simulink model "qam_model"  (R2013a)
settings: Solver=ode45  StartTime=0.0  StopTime=4e5*Tclk  RelTol=1e-3
PreLoadFcn:
  | crec_init;
StopFcn:
  | %offset = 70000;
  | % figure; u=sd(offset:end,:);plot(u(:,1)+j*u(:,2), '.');
values from neighbouring files (symbols this model uses):
  Fadc = 50    [qam_init.m]
  qam_mode = 2    [qam_init.m]
  Tclk = 1/Fclk    (= 0.01)    [qam_init.m]
undefined symbols (not defined in the file or in its folder): A, get, N
libraries: xbsIndex_r4 x29, commsink2 x7, dspsigops x3, dspsrcs4 x2, PPEthernetRuntimeCosim_r4 x1
settings Model: Creator=alexp  LastModifiedBy=diego
settings DataIOCC: MaxDataPoints=10000  SignalLoggingSaveFormat=ModelDataLogs
settings OptimizationCC: BooleanDataType=off  ExpressionDepthLimit=2147483647
settings DebuggingCC: SaveWithParameterizedLinksMsg=none  SignalResolutionControl=TryResolveAllWithWarning  SolverPrmCheckMsg=none  MultiTaskDSMMsg=warning  MultiTaskCondExecSysMsg=none  FcnCallInpInsideContextMsg=UseLocalSettings  StrictBusMsg=None
settings HardwareCC: TargetUnknown=on
settings RTWCC: IncludeERTFirstTime=on
settings GRTTargetCC: CombineOutputUpdateFcns=off  GRTInterface=on

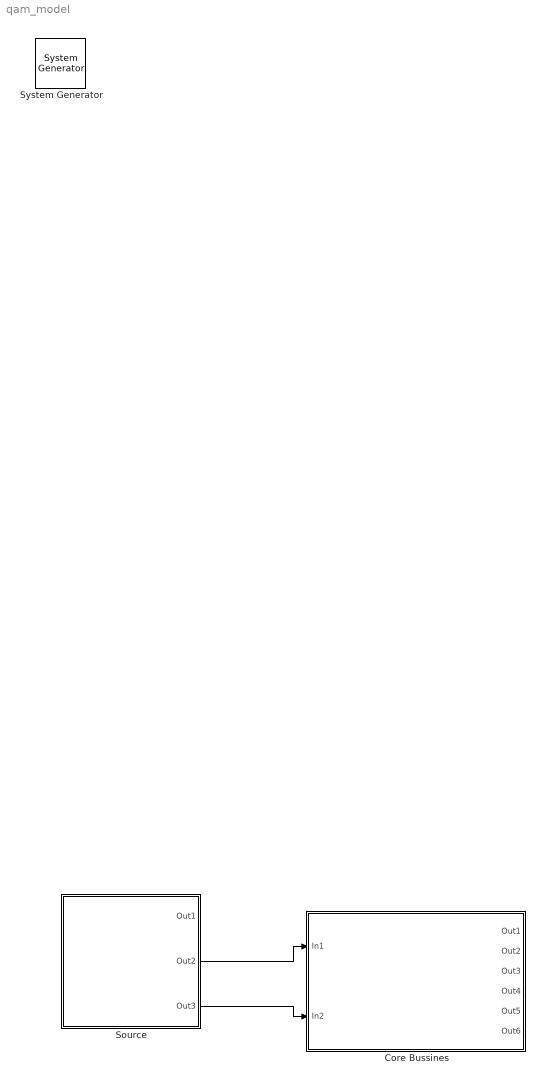
== system qam_model ==
  " System Generator" : xbsIndex_r4/ System Generator  Tag=genX  xilinxfamily=spartan6  part=xc6slx45t  speed=-3  package=fgg484  synthesis_tool=XST  clock_wrapper=Clock Enables  directory=./netlist  proj_type=Project Navigator  Synth_file=XST Defaults  Impl_file=ISE Defaults  testbench=off  simulink_period=Tclk  sysclk_period=20  dcm_input_clock_period=10  incr_netlist=off  trim_vbits=Everywhere in SubSystem  dbl_ovrd=According to Block Masks  core_generation=According to Block Masks  run_coregen=off  deprecated_control=off  eval_field=0  block_type=sysgen
  Core Bussines : Subsystem
  Source : Subsystem
  wires:
  Source/2(Out2) -> Core Bussines/1(In1)
  Source/3(Out3) -> Core Bussines/2(In2)

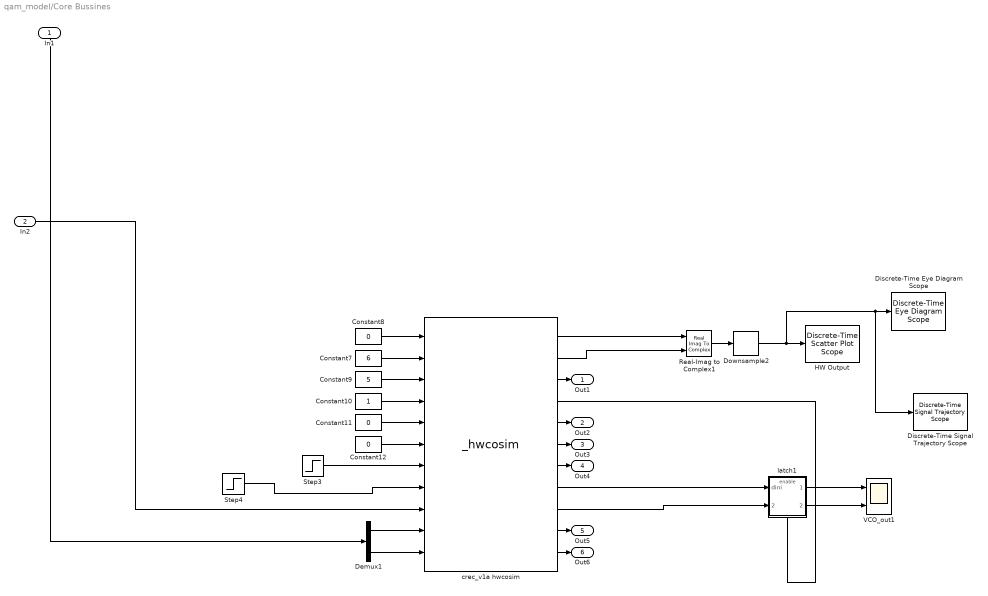
== system qam_model/Core Bussines ==
  In1 : Inport
  In2 : Inport  Port=2
  Constant10 : Constant
  Constant11 : Constant  Value=0
  Constant12 : Constant  Value=0
  Constant7 : Constant  Value=6
  Constant8 : Constant  Value=0
  Constant9 : Constant  Value=5
  Demux1 : Demux  Outputs=2
  Discrete-Time Eye Diagram Scope : commsink2/Discrete-Time Eye Diagram Scope  Tag=EyeDiagram  sampPerSymb=8  offsetEye=0  symbPerTrace=1  numTraces=800  numNewFrames=800  LineStyles=-  LineColors=[1 0 1]  dupPoints=on  fading=on  render=on  AxisGrid=on  yMin=-0.368939208984375  yMax=0.366009521484375  inphaseLabel=In-phase Amplitude  quadratureLabel=Quadrature Amplitude  openScopeAtSimStart=on  dispDiagram=In-phase and Quadrature  FrameNumber=off  FigPos=get(0,'defaultfigureposition');  figTitle=Eye Diagram  block_type_=eye  numLinesMax=8
  Discrete-Time Signal Trajectory Scope : commsink2/Discrete-Time Signal Trajectory Scope  Tag=SignalTrajectory  sampPerSymb=8  offsetEye=0  numTraces=800  numNewFrames=800  LineStyles=-  LineColors=b  fading=on  render=on  AxisGrid=on  xMin=-0.367013549804688  xMax=0.366525268554688  yMin=-0.368905639648438  yMax=0.364633178710938  inphaseLabel=In-phase Amplitude  quadratureLabel=Quadrature Amplitude  openScopeAtSimStart=on  FrameNumber=off  FigPos=get(0,'defaultfigureposition');  figTitle=Signal Trajectory  numLinesMax=8  block_type_=xy
  Downsample2 : dspsigops/Downsample  N=4  phase=0  InputProcessing=Columns as channels (frame based)  RateOptions=Allow multirate processing  smode=Allow multirate  fmode=Maintain input frame size  ic=0
  HW Output : commsink2/Discrete-Time Scatter Plot Scope  Tag=ScatterPlot  sampPerSymb=1  offsetEye=0  numTraces=2^qam_mode*1000  numNewFrames=2^qam_mode*200  LineMarkers=.  LineColors=[1 0 0]  fading=on  render=on  AxisGrid=on  xMin=-0.361343383789062  xMax=0.357070922851562  yMin=-0.360366821289062  yMax=0.358047485351562  inphaseLabel=In-phase Amplitude  quadratureLabel=Quadrature Amplitude  openScopeAtSimStart=on  FrameNumber=off  FigPos=get(0,'defaultfigureposition');  figTitle=Scatter Plot  numLinesMax=8  block_type_=scatter
  Real-Imag to Complex1 : RealImagToComplex
  Step3 : Step  Time=20*Tclk  Before=1  After=0  SampleTime=Tclk
  Step4 : Step  Time=100*Tclk  Before=1  After=0  SampleTime=Tclk
  VCO_out1 : Scope  NumInputPorts=2
      settings: YMin=-1~-1  YMax=1~1  SaveName=aa
  crec_v1a hwcosim : PPEthernetRuntimeCosim_r4/_hwcosim  clkSrc=Single Stepped  hasCombinationalPath=on  bitfileName=/home/diego/qam_demudulator/mirror/xapp1173/netlist/crec_v1a_cw.bit  ethernetInterface=Please select an Ethernet interface  fpgaEthernetAddr=00:0a:35:11:22:33  cable=Auto Detect  speed=N/A  cablePort=N/A  configTimeout=3000  configProfile=Default settings  enable_codebug=on  design_xtable=|  cosim_xtable=|  ethernetInterfaceID=eth0  timeout=3000  useWaitBox=1  prgClkFreq=10  bscanPos=1  Scheme=Cosim  hasProc=0  skipConfig=0  block_type=ppethernet_cosim
      design_xtable=|
      | {
      |   'clkWrapper' => 'crec_v1a_cw',
      |   'clocksGcd' => 1,
      |   'device' => 'xc6slx45t-3fgg484',
      |   'ports' => {
      |     'cnotrol' => {
      |       'bd_port_index' => 0,
      |       'direction' => 'in',
      |       'icon_text' => 'cnotrol',
      |       'period' => 1,
      |       'sim_pause_trigger' => false,
      |       'type' => 'UFix_2_0',
      |       'width' => 2,
      |     },
      |     'cnotrol1' => {
      |       'bd_port_index' => 1,
      |       'direction' => 'in',
      |       'icon_text' => 'cnotrol1',
      |       'period' => 1,
      |       'sim_pause_trigger' => false,
      |       'type' => 'Fix_8_0',
      |       'width' => 8,
      |     },
      |     'cnotrol2' => {
      |       'bd_port_index' => 2,
      |       'direction' => 'in',
      |       'icon_text' => 'cnotrol2',
      |       'period' => 1,
      |       'sim_pause_trigger' => false,
      |       'type' => 'Fix_8_0',
      |       'width' => 8,
      |     },
      |     'cnotrol3' => {
      |       'bd_port_index' => 3,
      |       'direction' => 'in',
      |       'icon_text' => 'cnotrol3',
      |       'period' => 1,
      |       'sim_pause_trigger' => false,
      |       'type' => 'Fix_8_0',
      |       'width' => 8,
      |     },
      |     'cnotrol4' => {
      |       'bd_port_index' => 4,
      |       'direction' => 'in',
      |       'icon_text' => 'cnotrol4',
      |       'period' => 1,
      |       'sim_pause_trigger' => false,
      |       'type' => 'UFix_1_0',
      |       'width' => 1,
      |     },
      |     'cnotrol5' => {
      |       'bd_port_index' => 5,
      |       'direction' => 'in',
      |       'icon_text' => 'cnotrol5',
      |       'period' => 1,
      |       'sim_pause_trigger' => false,
      |       'type' => 'Fix_28_26',
      |       'width' => 28,
      |     },
      |     'cnotrol6' => {
      |       'bd_port_index' => 6,
      |       'direction' => 'in',
      |       'icon_text' => 'cnotrol6',
      |       'period' => 1,
      |       'sim_pause_trigger' => false,
      |       'type' => 'Bool',
      |       'width' => 1,
      |     },
      |     'cnotrol7' => {
      |       'bd_port_index' => 7,
      |       'direction' => 'in',
      |       'icon_text' => 'cnotrol7',
      |       'period' => 1,
      |       'sim_pause_trigger' => false,
      |       'type' => 'Bool',
      |       'width' => 1,
      |     },
      |     'cnotrol8' => {
      |       'bd_port_index' => 8,
      |       'direction' => 'in',
      |       'icon_text' => 'cnotrol8',
      |       'period' => 1,
      |       'sim_pause_trigger' => false,
      |       'type' => 'Bool',
      |       'width' => 1,
      |     },
      |     'din_i' => {
      |       'bd_port_index' => 9,
      |       'direction' => 'in',
      |       'icon_text' => 'din_i',
      |       'period' => 1,
      |       'sim_pause_trigger' => false,
      |       'type' => 'Fix_16_13',
      |       'width' => 16,
      |     },
      |     'din_q' => {
      |       'bd_port_index' => 10,
      |       'direction' => 'in',
      |       'icon_text' => 'din_q',
      |       'period' => 1,
      |       'sim_pause_trigger' => false,
      |       'type' => 'Fix_16_13',
      |       'width' => 16,
      |     },
      |     'gateway_out' => {
      |       'bd_port_index' => 0,
      |       'direction' => 'out',
      |       'icon_text' => 'Gateway Out',
      |       'period' => 1,
      |       'sim_pause_trigger' => false,
      |       'type' => 'Fix_16_13',
      |       'width' => 16,
      |     },
      |     'gateway_out1' => {
      |       'bd_port_index' => 1,
      |       'direction' => 'out',
      |       'icon_text' => 'Gateway Out1',
      |       'period' => 1,
      |       'sim_pause_trigger' => false,
      |       'type' => 'Fix_16_13',
      |       'width' => 16,
      |     },
      |     'gateway_out10' => {
      |       'bd_port_index' => 2,
      |       'direction' => 'out',
      |       'icon_text' => 'Gateway Out10',
      |       'period' => 1,
      |       'sim_pause_trigger' => false,
      |       'type' => 'Fix_12_11',
      |       'width' => 12,
      |     },
      |     'gateway_out2' => {
      |       'bd_port_index' => 3,
      |       'direction' => 'out',
      |       'icon_text' => 'Gateway Out2',
      |       'period' => 1,
      |       'sim_pause_trigger' => false,
      |       'type' => 'Bool',
      |       'width' => 1,
      |     },
      |     'gateway_out3' => {
      |       'bd_port_index' => 4,
      |       'direction' => 'out',
      |       'icon_text' => 'Gateway Out3',
      |       'period' => 1,
      |       'sim_pause_trigger' => false,
      |       'type' => 'Fix_28_26',
      |       'width' => 28,
      |     },
      |     'gateway_out4' => {
      |       'bd_port_index' => 5,
      |       'direction' => 'out',
      |       'icon_text' => 'Gateway Out4',
      |       'period' => 1,
      |       'sim_pause_trigger' => false,
      |       'type' => 'Bool',
      |       'width' => 1,
      |     },
      |     'gateway_out5' => {
      |       'bd_port_index' => 6,
      |       'direction' => 'out',
      |       'icon_text' => 'Gateway Out5',
      |       'period' => 1,
      |       'sim_pause_trigger' => false,
      |       'type' => 'Bool',
      |       'width' => 1,
      |     },
      |     'gateway_out6' => {
      |       'bd_port_index' => 7,
      |       'direction' => 'out',
      |       'icon_text' => 'Gateway Out6',
      |       'period' => 1,
      |       'sim_pause_trigger' => false,
      |       'type' => 'Fix_12_11',
      |       'width' => 12,
      |     },
      |     'gateway_out7' => {
      |       'bd_port_index' => 8,
      |       'direction' => 'out',
      |       'icon_text' => 'Gateway Out7',
      |       'period' => 1,
      |       'sim_pause_trigger' => false,
      |       'type' => 'Fix_12_11',
      |       'width' => 12,
      |     },
      |     'gateway_out8' => {
      |       'bd_port_index' => 9,
      |       'direction' => 'out',
      |       'icon_text' => 'Gateway Out8',
      |       'period' => 1,
      |       'sim_pause_trigger' => false,
      |       'type' => 'Bool',
      |       'width' => 1,
      |     },
      |     'gateway_out9' => {
      |       'bd_port_index' => 10,
      |       'direction' => 'out',
      |       'icon_text' => 'Gateway Out9',
      |       'period' => 1,
      |       'sim_pause_trigger' => false,
      |       'type' => 'Fix_12_11',
      |       'width' => 12,
      |     },
      |   },
      |   'shared_memories' => {},
      | }
      cosim_xtable=|
      | {
      |   'ethernetCosim' => {
      |     'blockRAMSize' => 2048,
      |     'bscanPos' => 2,
      |     'maxFrameSize' => 8184,
      |     'target' => 'sp605',
      |     'type' => 'ppethernet',
      |   },
      | }
  latch1 : Subsystem  TreatAsAtomicUnit=on
  Out1 : Outport
  Out2 : Outport  Port=2
  Out3 : Outport  Port=3
  Out4 : Outport  Port=4
  Out5 : Outport  Port=5
  Out6 : Outport  Port=6
  wires:
  Step3/1 -> crec_v1a hwcosim/7
  Step4/1 -> crec_v1a hwcosim/8
  Demux1/2 -> crec_v1a hwcosim/11
  Demux1/1 -> crec_v1a hwcosim/10
  Downsample2/1 -> Discrete-Time Signal Trajectory Scope/1, Discrete-Time Eye Diagram Scope/1, HW Output/1
  Real-Imag to Complex1/1 -> Downsample2/1
  crec_v1a hwcosim/8 -> latch1/1(dini)
  crec_v1a hwcosim/2 -> Real-Imag to Complex1/2
  crec_v1a hwcosim/1 -> Real-Imag to Complex1/1
  crec_v1a hwcosim/10 -> Out5/1
  crec_v1a hwcosim/7 -> Out4/1
  crec_v1a hwcosim/5 -> Out2/1
  In1/1 -> Demux1/1
  Constant11/1 -> crec_v1a hwcosim/5
  In2/1 -> crec_v1a hwcosim/9
  Constant8/1 -> crec_v1a hwcosim/1
  Constant9/1 -> crec_v1a hwcosim/3
  Constant10/1 -> crec_v1a hwcosim/4
  crec_v1a hwcosim/6 -> Out3/1
  crec_v1a hwcosim/11 -> Out6/1
  crec_v1a hwcosim/3 -> Out1/1
  crec_v1a hwcosim/4 -> latch1/Enable
  latch1/2(doutq) -> VCO_out1/2
  crec_v1a hwcosim/9 -> latch1/2(dinq)
  latch1/1(douti) -> VCO_out1/1
  Constant12/1 -> crec_v1a hwcosim/6
  Constant7/1 -> crec_v1a hwcosim/2

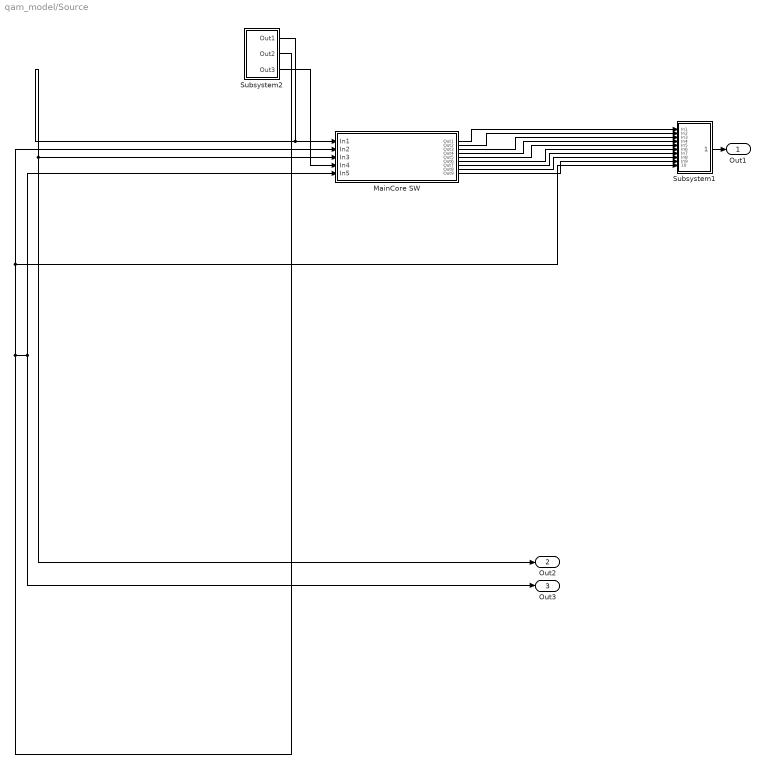
== system qam_model/Source ==
  MainCore SW : Subsystem
  Subsystem1 : Subsystem
  Subsystem2 : Subsystem
  Out1 : Outport
  Out2 : Outport  Port=2
  Out3 : Outport  Port=3
  wires:
  Subsystem2/3(Out3) -> MainCore SW/4(In4)
  Subsystem1/1(Out1) -> Out1/1
  MainCore SW/5(Out5) -> Subsystem1/5(In5)
  MainCore SW/3(Out3) -> Subsystem1/3(In3)
  Subsystem2/2(Out2) -> MainCore SW/2(In2), Subsystem1/10(In10), Out3/1, MainCore SW/5(In5)
  MainCore SW/8(Out8) -> Subsystem1/8(In8)
  MainCore SW/2(Out2) -> Subsystem1/2(In2)
  MainCore SW/4(Out4) -> Subsystem1/4(In4)
  Subsystem2/1(Out1) -> Out2/1, MainCore SW/3(In3), MainCore SW/1(In1)
  MainCore SW/9(Out9) -> Subsystem1/9(In9)
  MainCore SW/6(Out6) -> Subsystem1/6(In6)
  MainCore SW/7(Out7) -> Subsystem1/7(In7)
  MainCore SW/1(Out1) -> Subsystem1/1(In1)

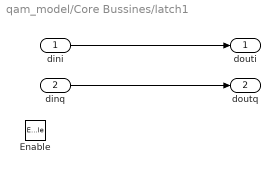
== system qam_model/Core Bussines/latch1 ==
  dini : Inport
  dinq : Inport  Port=2
  Enable : EnablePort
  douti : Outport
  doutq : Outport  Port=2
  wires:
  dini/1 -> douti/1
  dinq/1 -> doutq/1

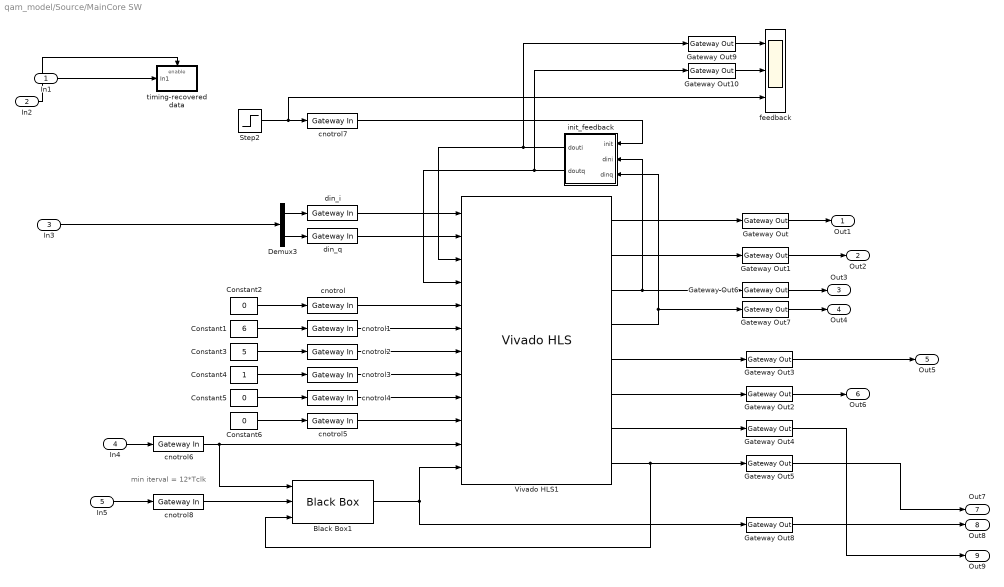
== system qam_model/Source/MainCore SW ==
  note: min iterval = 12*Tclk
  In1 : Inport
  In2 : Inport  Port=2
  In3 : Inport  Port=3
  In4 : Inport  Port=4
  In5 : Inport  Port=5
  Black Box1 : xbsIndex_r4/Black Box  init_code=start_config  sim_method=ISE Simulator  verbose=off  block_type=blackbox2
  Constant1 : Constant  Value=6
  Constant2 : Constant  Value=0
  Constant3 : Constant  Value=5
  Constant4 : Constant
  Constant5 : Constant  Value=0
  Constant6 : Constant  Value=0
  Demux3 : Demux  Outputs=2
  Gateway Out{,1..10} (11 alike) : xbsIndex_r4/Gateway Out  inherit_from_input=off  hdl_port=on  timing_constraint=None  locs_specified=off  LOCs={}  UseAsDAC=off  DACChannel='1'  block_type=gatewayout
  Step2 : Step  Time=100*Tclk  Before=1  After=0  SampleTime=Tclk
  Vivado HLS1 : xbsIndex_r4/Vivado HLS  anytable='/home/diego/qam_demudulator/mirror/xapp1173/VHLS_proj/sol3_dataflow_io/'  display_datatype=off  rate_propagation_method=Simulink system period  model_file_path=''  latency=1  block_type=hls
      settings: infoedit=This block allows including C,C++ and SystemC source files in System Generator for DSP designs.
  cnotrol : xbsIndex_r4/Gateway In  gui_display_data_type=Fixed-point  arith_type=Unsigned  n_bits=2  bin_pt=0  preci_type=Single  exp_width=8  frac_width=24  quantization=Truncate  overflow=Wrap  period=Tclk  dbl_ovrd=off  timing_constraint=None  locs_specified=off  LOCs={}  UseAsADC=off  ADCChannel='1'  inherit_from_input=off  hdl_port=on  block_type=gatewayin
  cnotrol1 : xbsIndex_r4/Gateway In  gui_display_data_type=Fixed-point  arith_type="Signed  (2's comp)"  n_bits=8  bin_pt=0  preci_type=Single  exp_width=8  frac_width=24  quantization=Truncate  overflow=Wrap  period=Tclk  dbl_ovrd=off  timing_constraint=None  locs_specified=off  LOCs={}  UseAsADC=off  ADCChannel='1'  inherit_from_input=off  hdl_port=on  block_type=gatewayin
  cnotrol2 : xbsIndex_r4/Gateway In  gui_display_data_type=Fixed-point  arith_type="Signed  (2's comp)"  n_bits=8  bin_pt=0  preci_type=Single  exp_width=8  frac_width=24  quantization=Truncate  overflow=Wrap  period=Tclk  dbl_ovrd=off  timing_constraint=None  locs_specified=off  LOCs={}  UseAsADC=off  ADCChannel='1'  inherit_from_input=off  hdl_port=on  block_type=gatewayin
  cnotrol3 : xbsIndex_r4/Gateway In  gui_display_data_type=Fixed-point  arith_type="Signed  (2's comp)"  n_bits=8  bin_pt=0  preci_type=Single  exp_width=8  frac_width=24  quantization=Truncate  overflow=Wrap  period=Tclk  dbl_ovrd=off  timing_constraint=None  locs_specified=off  LOCs={}  UseAsADC=off  ADCChannel='1'  inherit_from_input=off  hdl_port=on  block_type=gatewayin
  cnotrol4 : xbsIndex_r4/Gateway In  gui_display_data_type=Fixed-point  arith_type=Unsigned  n_bits=1  bin_pt=0  preci_type=Single  exp_width=8  frac_width=24  quantization=Truncate  overflow=Wrap  period=Tclk  dbl_ovrd=off  timing_constraint=None  locs_specified=off  LOCs={}  UseAsADC=off  ADCChannel='1'  inherit_from_input=off  hdl_port=on  block_type=gatewayin
  cnotrol5 : xbsIndex_r4/Gateway In  gui_display_data_type=Fixed-point  arith_type="Signed  (2's comp)"  n_bits=28  bin_pt=26  preci_type=Single  exp_width=8  frac_width=24  quantization=Truncate  overflow=Wrap  period=Tclk  dbl_ovrd=off  timing_constraint=None  locs_specified=off  LOCs={}  UseAsADC=off  ADCChannel='1'  inherit_from_input=off  hdl_port=on  block_type=gatewayin
  cnotrol6 : xbsIndex_r4/Gateway In  gui_display_data_type=Boolean  arith_type=Boolean  n_bits=2  bin_pt=0  preci_type=Single  exp_width=8  frac_width=24  quantization=Truncate  overflow=Wrap  period=Tclk  dbl_ovrd=off  timing_constraint=None  locs_specified=off  LOCs={}  UseAsADC=off  ADCChannel='1'  inherit_from_input=off  hdl_port=on  block_type=gatewayin
  cnotrol7 : xbsIndex_r4/Gateway In  gui_display_data_type=Boolean  arith_type=Boolean  n_bits=2  bin_pt=0  preci_type=Single  exp_width=8  frac_width=24  quantization=Truncate  overflow=Wrap  period=Tclk  dbl_ovrd=off  timing_constraint=None  locs_specified=off  LOCs={}  UseAsADC=off  ADCChannel='1'  inherit_from_input=off  hdl_port=on  block_type=gatewayin
  cnotrol8 : xbsIndex_r4/Gateway In  gui_display_data_type=Boolean  arith_type=Boolean  n_bits=2  bin_pt=0  preci_type=Single  exp_width=8  frac_width=24  quantization=Truncate  overflow=Wrap  period=Tclk  dbl_ovrd=off  timing_constraint=None  locs_specified=off  LOCs={}  UseAsADC=off  ADCChannel='1'  inherit_from_input=off  hdl_port=on  block_type=gatewayin
  din_i : xbsIndex_r4/Gateway In  gui_display_data_type=Fixed-point  arith_type="Signed  (2's comp)"  n_bits=16  bin_pt=13  preci_type=Single  exp_width=8  frac_width=24  quantization=Truncate  overflow=Wrap  period=Tclk  dbl_ovrd=off  timing_constraint=None  locs_specified=off  LOCs={}  UseAsADC=off  ADCChannel='1'  inherit_from_input=off  hdl_port=on  block_type=gatewayin
  din_q : xbsIndex_r4/Gateway In  gui_display_data_type=Fixed-point  arith_type="Signed  (2's comp)"  n_bits=16  bin_pt=13  preci_type=Single  exp_width=8  frac_width=24  quantization=Truncate  overflow=Wrap  period=Tclk  dbl_ovrd=off  timing_constraint=None  locs_specified=off  LOCs={}  UseAsADC=off  ADCChannel='1'  inherit_from_input=off  hdl_port=on  block_type=gatewayin
  feedback : Scope  NumInputPorts=3
      settings: YMin=-1~-1~-5  YMax=1~1~5  SaveName=aa1
  init_feedback : Subsystem
  timing-recovered data : Subsystem  TreatAsAtomicUnit=on
  Out1 : Outport
  Out2 : Outport  Port=2
  Out3 : Outport  Port=3
  Out4 : Outport  Port=4
  Out5 : Outport  Port=5
  Out6 : Outport  Port=6
  Out7 : Outport  Port=7
  Out8 : Outport  Port=8
  Out9 : Outport  Port=9
  wires:
  In5/1 -> cnotrol8/1
  In2/1 -> timing-recovered data/Enable
  In1/1 -> timing-recovered data/1(In1)
  Constant3/1 -> cnotrol2/1
  Constant2/1 -> cnotrol/1
  Constant1/1 -> cnotrol1/1
  Constant4/1 -> cnotrol3/1
  Constant5/1 -> cnotrol4/1
  Constant6/1 -> cnotrol5/1
  In4/1 -> cnotrol6/1
  Demux3/2 -> din_q/1
  Demux3/1 -> din_i/1
  Gateway Out3/1 -> Out5/1
  cnotrol/1 -> Vivado HLS1/5
  cnotrol1/1 -> Vivado HLS1/6
  cnotrol2/1 -> Vivado HLS1/7
  cnotrol3/1 -> Vivado HLS1/8
  cnotrol4/1 -> Vivado HLS1/9
  cnotrol5/1 -> Vivado HLS1/10
  cnotrol6/1 -> Vivado HLS1/11, Black Box1/1
  din_i/1 -> Vivado HLS1/1
  din_q/1 -> Vivado HLS1/2
  Vivado HLS1/1 -> Gateway Out/1
  Vivado HLS1/2 -> Gateway Out1/1
  Vivado HLS1/5 -> Gateway Out3/1
  Vivado HLS1/6 -> Gateway Out2/1
  Vivado HLS1/7 -> Gateway Out4/1
  Vivado HLS1/8 -> Gateway Out5/1, Black Box1/3
  Gateway Out4/1 -> Out9/1
  cnotrol8/1 -> Black Box1/2
  Black Box1/1 -> Vivado HLS1/12, Gateway Out8/1
  Gateway Out2/1 -> Out6/1
  Gateway Out/1 -> Out1/1
  Gateway Out1/1 -> Out2/1
  Gateway Out5/1 -> Out7/1
  init_feedback/1(douti) -> Gateway Out9/1, Vivado HLS1/3
  init_feedback/2(doutq) -> Gateway Out10/1, Vivado HLS1/4
  Vivado HLS1/4 -> init_feedback/3(dinq), Gateway Out7/1
  Vivado HLS1/3 -> init_feedback/2(dini), Gateway Out6/1
  Step2/1 -> cnotrol7/1, feedback/3
  cnotrol7/1 -> init_feedback/1(init)
  Gateway Out6/1 -> Out3/1
  Gateway Out7/1 -> Out4/1
  Gateway Out8/1 -> Out8/1
  Gateway Out9/1 -> feedback/1
  Gateway Out10/1 -> feedback/2
  In3/1 -> Demux3/1

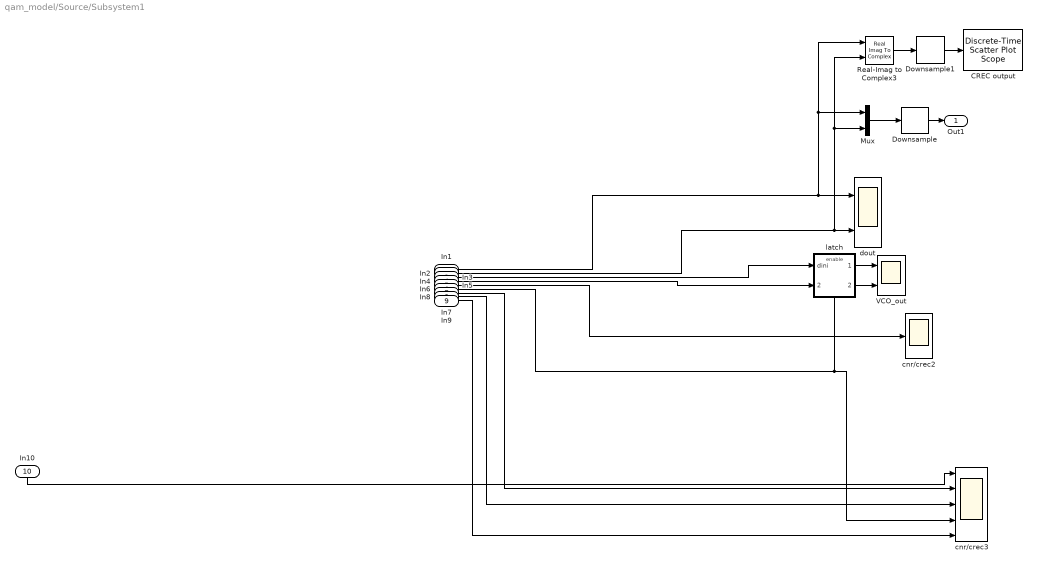
== system qam_model/Source/Subsystem1 ==
  In1 : Inport
  In2 : Inport  Port=2
  In3 : Inport  Port=3
  In4 : Inport  Port=4
  In5 : Inport  Port=5
  In6 : Inport  Port=6
  In7 : Inport  Port=7
  In8 : Inport  Port=8
  In9 : Inport  Port=9
  In10 : Inport  Port=10
  CREC output : commsink2/Discrete-Time Scatter Plot Scope  Tag=ScatterPlot  sampPerSymb=1  offsetEye=0  numTraces=2^qam_mode*1000  numNewFrames=2^qam_mode*200  LineMarkers=.  LineColors=b  fading=on  render=on  AxisGrid=on  xMin=-1.2  xMax=1.2  yMin=-1.2  yMax=1.2  inphaseLabel=In-phase Amplitude  quadratureLabel=Quadrature Amplitude  openScopeAtSimStart=on  FrameNumber=off  FigPos=get(0,'defaultfigureposition');  figTitle=Scatter Plot  numLinesMax=8  block_type_=scatter
  Downsample : dspsigops/Downsample  N=4  phase=0  InputProcessing=Columns as channels (frame based)  RateOptions=Allow multirate processing  smode=Allow multirate  fmode=Maintain input frame size  ic=0
  Downsample1 : dspsigops/Downsample  N=4  phase=0  InputProcessing=Columns as channels (frame based)  RateOptions=Allow multirate processing  smode=Allow multirate  fmode=Maintain input frame size  ic=0
  Mux : Mux  Inputs=2
  Real-Imag to Complex3 : RealImagToComplex
  VCO_out : Scope  NumInputPorts=2
      settings: YMin=-1~-1  YMax=1~1  SaveName=aa9
  cnr/crec2 : Scope
      settings: TimeRange=4000  YMin=-0.0012  YMax=0.0004  SaveName=aa6  Decimation=32
  cnr/crec3 : Scope  NumInputPorts=5
      settings: YMin=0~0~0~0~0  YMax=1.2~1.1~1.2~1.2~1.2  SaveName=aa7
  dout : Scope  NumInputPorts=2
      settings: YMin=-0.4~-0.4  YMax=0.4~0.4  SaveName=aa8
  latch : Subsystem  TreatAsAtomicUnit=on
  Out1 : Outport
  wires:
  In2/1 -> dout/2, Mux/2, Real-Imag to Complex3/2
  In1/1 -> Mux/1, Real-Imag to Complex3/1, dout/1
  In10/1 -> cnr/crec3/1
  In3/1 -> latch/1(dini)
  In7/1 -> cnr/crec3/2
  In9/1 -> cnr/crec3/5
  Downsample/1 -> Out1/1
  In5/1 -> cnr/crec2/1
  In8/1 -> cnr/crec3/3
  In4/1 -> latch/2(dinq)
  Mux/1 -> Downsample/1
  Real-Imag to Complex3/1 -> Downsample1/1
  Downsample1/1 -> CREC output/1
  latch/1(douti) -> VCO_out/1
  latch/2(doutq) -> VCO_out/2
  In6/1 -> latch/Enable, cnr/crec3/4

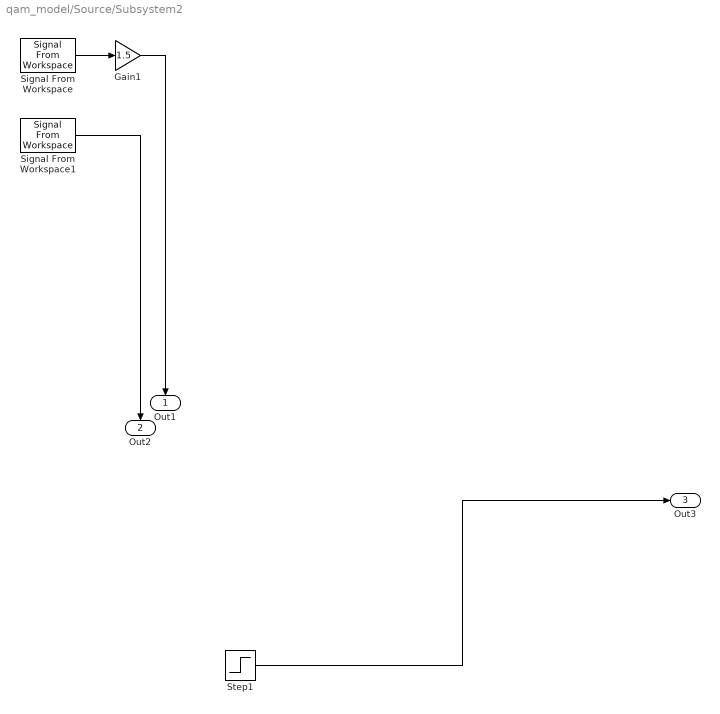
== system qam_model/Source/Subsystem2 ==
  Gain1 : Gain  Gain=1.5
  Signal From Workspace : dspsrcs4/Signal From Workspace  X=cinput  Ts=2/Fadc  nsamps=1  OutputAfterFinalValue=Setting to zero  ignoreOrWarnInputAndFrameLengths=off
  Signal From Workspace1 : dspsrcs4/Signal From Workspace  X=en1x  Ts=2/Fadc  nsamps=1  OutputAfterFinalValue=Setting to zero  ignoreOrWarnInputAndFrameLengths=off
  Step1 : Step  Time=20*Tclk  Before=1  After=0  SampleTime=Tclk
  Out1 : Outport
  Out2 : Outport  Port=2
  Out3 : Outport  Port=3
  wires:
  Step1/1 -> Out3/1
  Signal From Workspace/1 -> Gain1/1
  Signal From Workspace1/1 -> Out2/1
  Gain1/1 -> Out1/1

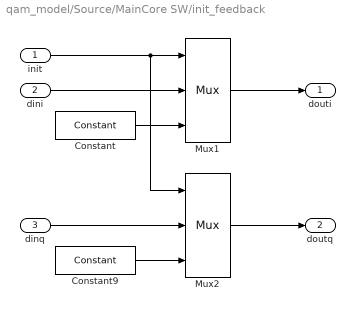
== system qam_model/Source/MainCore SW/init_feedback ==
  init : Inport
  dini : Inport  Port=2
  dinq : Inport  Port=3
  Constant : xbsIndex_r4/Constant  const=1  gui_display_data_type=Fixed-point  arith_type=Signed (2's comp)  n_bits=12  bin_pt=11  preci_type=Single  exp_width=8  frac_width=24  explicit_period=off  period=1  equ=P=C  opselect=C  inp2=PCIN>>17  opr=+  inp1=P  carry=CIN  dbl_ovrd=off  block_type=constant
  Constant9 : xbsIndex_r4/Constant  const=0  gui_display_data_type=Fixed-point  arith_type=Signed (2's comp)  n_bits=12  bin_pt=11  preci_type=Single  exp_width=8  frac_width=24  explicit_period=off  period=1  equ=P=C  opselect=C  inp2=PCIN>>17  opr=+  inp1=P  carry=CIN  dbl_ovrd=off  block_type=constant
  Mux1 : xbsIndex_r4/Mux  inputs=2  en=off  latency=1  precision=Full  arith_type=Unsigned  n_bits=16  bin_pt=14  quantization=Truncate  overflow=Wrap  dbl_ovrd=off  block_type=mux
  Mux2 : xbsIndex_r4/Mux  inputs=2  en=off  latency=1  precision=Full  arith_type=Unsigned  n_bits=16  bin_pt=14  quantization=Truncate  overflow=Wrap  dbl_ovrd=off  block_type=mux
  douti : Outport
  doutq : Outport  Port=2
  wires:
  Constant/1 -> Mux1/3
  Constant9/1 -> Mux2/3
  init/1 -> Mux1/1, Mux2/1
  dini/1 -> Mux1/2
  dinq/1 -> Mux2/2
  Mux1/1 -> douti/1
  Mux2/1 -> doutq/1

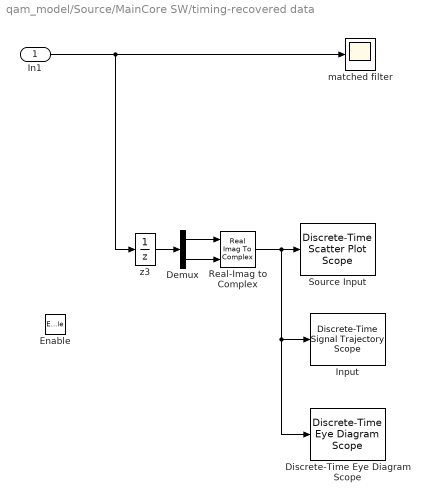
== system qam_model/Source/MainCore SW/timing-recovered data ==
  In1 : Inport
  Enable : EnablePort
  Demux : Demux  Outputs=2
  Discrete-Time Eye Diagram Scope : commsink2/Discrete-Time Eye Diagram Scope  Tag=EyeDiagram  sampPerSymb=8  offsetEye=0  symbPerTrace=1  numTraces=800  numNewFrames=800  LineStyles=-  LineColors=b  dupPoints=on  fading=on  render=on  AxisGrid=on  yMin=-3.15  yMax=3.15  inphaseLabel=In-phase Amplitude  quadratureLabel=Quadrature Amplitude  openScopeAtSimStart=on  dispDiagram=In-phase and Quadrature  FrameNumber=off  FigPos=get(0,'defaultfigureposition');  figTitle=Eye Diagram  block_type_=eye  numLinesMax=8
  "Input " : commsink2/Discrete-Time Signal Trajectory Scope  Tag=SignalTrajectory  sampPerSymb=8  offsetEye=0  numTraces=800  numNewFrames=800  LineStyles=-  LineColors=b  fading=on  render=on  AxisGrid=on  xMin=-3.3  xMax=3.315  yMin=-3.3  yMax=3.315  inphaseLabel=In-phase Amplitude  quadratureLabel=Quadrature Amplitude  openScopeAtSimStart=on  FrameNumber=off  FigPos=get(0,'defaultfigureposition');  figTitle=Signal Trajectory  numLinesMax=8  block_type_=xy
  Real-Imag to Complex : RealImagToComplex
  "Source Input " : commsink2/Discrete-Time Scatter Plot Scope  Tag=ScatterPlot  sampPerSymb=1  offsetEye=0  numTraces=800  numNewFrames=100  LineMarkers=.  LineColors=[1 0 0]  fading=on  render=on  AxisGrid=on  xMin=-0.567681884765625  xMax=0.611260986328125  yMin=-0.583612060546875  yMax=0.595330810546875  inphaseLabel=In-phase Amplitude  quadratureLabel=Quadrature Amplitude  openScopeAtSimStart=on  FrameNumber=off  FigPos=get(0,'defaultfigureposition');  figTitle=Scatter Plot  numLinesMax=8  block_type_=scatter
  matched filter : Scope
      settings: YMin=0  YMax=70  SaveName=ScopeData7  Decimation=32
  z3 : UnitDelay  SampleTime=-1
  wires:
  z3/1 -> Demux/1
  In1/1 -> matched filter/1, z3/1
  Demux/1 -> Real-Imag to Complex/1
  Demux/2 -> Real-Imag to Complex/2
  Real-Imag to Complex/1 -> Discrete-Time Eye Diagram Scope/1, "Input "/1, "Source Input "/1

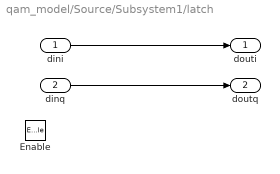
== system qam_model/Source/Subsystem1/latch ==
  dini : Inport
  dinq : Inport  Port=2
  Enable : EnablePort
  douti : Outport
  doutq : Outport  Port=2
  wires:
  dini/1 -> douti/1
  dinq/1 -> doutq/1
